simulink model "Filtered_Signal"  (R2023a)
settings: Solver=VariableStepAuto  StartTime=0.0  StopTime=10.0  RelTol=1e-3
settings Model: Creator=Aman  LastModifiedBy=Aman

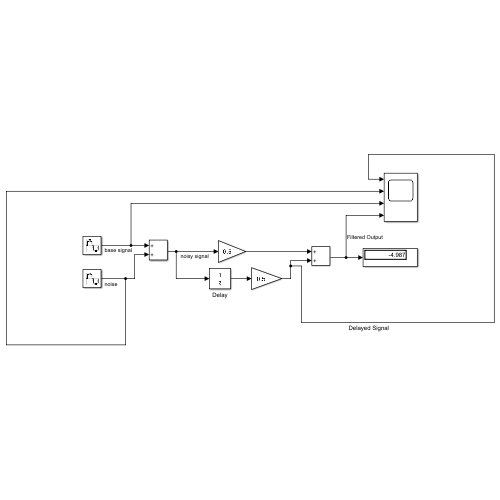
[thumbnail: Simulink's stored preview of the top-level diagram]
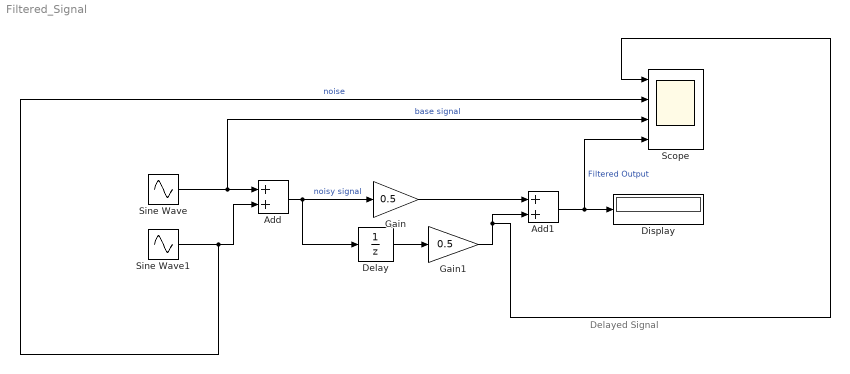
== system Filtered_Signal ==
  note: Delayed Signal
  Add : Sum
  Add1 : Sum
  Delay : UnitDelay  SampleTime=.2  HasFrameUpgradeWarning=on
  Display : Display
  Gain : Gain  Gain=0.5
  Gain1 : Gain  Gain=0.5
  Scope : Scope  NumInputPorts=4
  Sine Wave : Sin  Amplitude=10  SampleTime=.2
  Sine Wave1 : Sin  Amplitude=2.5  Frequency=18  SampleTime=.2
  wires:
  Add1/1 -> Scope/4, Display/1  "Filtered Output"
  Sine Wave1/1 -> Add/2, Scope/2  "noise"
  Gain/1 -> Add1/1
  Add/1 -> Gain/1, Delay/1  "noisy signal"
  Delay/1 -> Gain1/1
  Sine Wave/1 -> Scope/3, Add/1  "base signal"
  Gain1/1 -> Scope/1, Add1/2
